simulink model "Model_6DOF_dk"  (R2022a)
settings: Solver=FixedStepAuto  StartTime=0.0  StopTime=Tf  FixedStep=0.05  RelTol=1e-3
InitFcn:
  | run;
StopFcn:
  | save('testdata')
values from neighbouring files (symbols this model uses):
  adap = 1    [run.m]    (also in testdata.mat)
  Ba_0 = [0 0 0 0 0 0]    [run.m]    (also in testdata.mat)
  Bb = 4418825.3321    [testdata.mat]
  Bv_0 = [-5.14444 0 0 0 0 0]    [run.m]    (also in testdata.mat)
  Bx_0 = [0 0 -12 0 0 0]    [run.m]    (also in testdata.mat)
  dA_BP1 = [0.00388591051125 0.00354364911083 0.00553040741788 0.00502167988714 0.0078585088908 0.00748424955325 0.0119232766011 0.0109054787122 0.0168329706434 0.016985509009 0.0156802934897 0.014556760782 ... (616 elements, 616x1)]    [testdata.mat]
  dA_BP2 = [0.00388594063171 0.00354357191533 0.00553040491113 0.00502170939051 0.00785855989083 0.00748435285791 0.0119232653011 0.0109054419481 0.0168329955973 0.0169854794658 0.015680230324 0.0145567225609 ... (616 elements, 616x1)]    [testdata.mat]
  dA_Hull = [0.896301676511 0.898896720864 0.884294141897 0.886832830172 0.870887902011 0.873360353662 0.856223658523 0.858613244346 0.840314828191 0.842595287849 0.823129385532 0.8253007603 ... (2914 elements, 2914x1)]    [testdata.mat]
  dA_PH = [0.00917454029683 0.00917454029683 0.00646521761836 0.00644666811643 0.011728531678 0.0107683420972 0.0165186720105 0.0100399866209 0.0121147162203 0.00917369783051 0.00917369783051 0.00646462373197 ... (550 elements, 550x1)]    [testdata.mat]
  dA_Sail = [0.08073747293 0.0655437895785 0.0678199581962 0.211496702297 0.185444652254 0.10949647106 0.0763960001413 0.0735864235671 0.0440728222699 0.281106392154 0.32735958292 0.104041938486 ... (564 elements, 564x1)]    [testdata.mat]
  dA_SProot = [0.0225345452169 0.0247277274893 0.0225345452169 0.0480467976325 0.0166447079844 0.0410754287554 0.0247277274893 0.0480467976325 0.0468898715351 0.0839833312794 0.0166447079844 0.0255016718 ... (904 elements, 904x1)]    [testdata.mat]
  dA_X1a = [0.0149621011817 0.0166706156701 0.0341149781095 0.0355915100668 0.0512235531199 0.0489176133683 0.0604458424392 0.0503279152264 0.0577124835488 0.0401555322121 0.044833653096 0.0251568218541 ... (200 elements, 200x1)]    [testdata.mat]
  dA_X1b = [0.0149621011817 0.0166706156701 0.0341149781095 0.0355915100668 0.0512235531199 0.0489176133683 0.0604458424392 0.0503279152264 0.0577124835488 0.0401555322121 0.044833653096 0.0251568218541 ... (200 elements, 200x1)]    [testdata.mat]
  dA_X2a = [0.0149620639393 0.0166705502855 0.0341150948266 0.0355913495849 0.051223110376 0.0489180393921 0.0604458270347 0.0503275686692 0.0577128112225 0.0401556683139 0.0448334591683 0.0251566482124 ... (200 elements, 200x1)]    [testdata.mat]
  dA_X2b = [0.0149620639393 0.0166705502855 0.0341150948266 0.0355913495849 0.051223110376 0.0489180393921 0.0604458270347 0.0503275686692 0.0577128112225 0.0401556683139 0.0448334591683 0.0251566482124 ... (200 elements, 200x1)]    [testdata.mat]
  dA_X3a = [0.0149621011817 0.0166706156701 0.0341149781095 0.0355915100668 0.0512235531199 0.0489176133683 0.0604458424392 0.0503279152264 0.0577124835488 0.0401555322121 0.044833653096 0.0251568218541 ... (200 elements, 200x1)]    [testdata.mat]
  dA_X3b = [0.0149621011817 0.0166706156701 0.0341149781095 0.0355915100668 0.0512235531199 0.0489176133683 0.0604458424392 0.0503279152264 0.0577124835488 0.0401555322121 0.044833653096 0.0251568218541 ... (200 elements, 200x1)]    [testdata.mat]
  dA_X4a = [0.0149621011817 0.0166706156701 0.0341149781095 0.0355915100668 0.0512235531199 0.0489176133683 0.0604458424392 0.0503279152264 0.0577124835488 0.0401555322121 0.044833653096 0.0251568218541 ... (200 elements, 200x1)]    [testdata.mat]
  dA_X4b = [0.0149621011817 0.0166706156701 0.0341149781095 0.0355915100668 0.0512235531199 0.0489176133683 0.0604458424392 0.0503279152264 0.0577124835488 0.0401555322121 0.044833653096 0.0251568218541 ... (200 elements, 200x1)]    [testdata.mat]
  Ixx = 52300000    [testdata.mat]
  Ixy = 0    [testdata.mat]
  Ixz = 0    [testdata.mat]
  Iyy = 1375000000    [testdata.mat]
  Iyz = 0    [testdata.mat]
  Izz = 1367000000    [testdata.mat]
  L1 =     [testdata.mat]
  Mb = 4418825.3321    [testdata.mat]
  n_BP1 = [-0.7747315 -0.03638153 -0.4095958 0 -0.1221389 0 -0.01670914 0 0.005209626 0 0.03404154 0 ... (1848 elements, 616x3)]    [testdata.mat]
  n_BP2 = [-0.774731517 -0.0363815315 -0.409595788 0 -0.122138903 0 -0.0167091396 0 0.00520962616 0 0.0340415388 0 ... (1848 elements, 616x3)]    [testdata.mat]
  n_Hull = [-3.334458e-05 -1.700098e-14 -3.354233e-05 -1.686235e-14 -3.289162e-05 -1.685701e-14 -3.291391e-05 -1.698144e-14 -3.338145e-05 -1.688959e-14 -3.29289e-05 -1.682536e-14 ... (8742 elements, 2914x3)]    [testdata.mat]
  n_PH = [0 0 0.01711651 0.01711627 0.2676807 0.2676804 0.7675173 0.7675174 0.9857236 0 0 0.01711456 ... (1650 elements, 550x3)]    [testdata.mat]
  n_Sail = [-0.05126832 -0.05168081 -0.0485872 -0.03288998 -0.03203588 -0.04435105 -0.04335441 -0.04419429 -0.05169604 0.01094904 0.01649325 -0.03825178 ... (1692 elements, 564x3)]    [testdata.mat]
  n_SProot = [-0.7837688 -0.7969784 -0.7837688 -0.79448 -0.280412 -0.3378876 -0.7969784 -0.79448 -0.7910827 -0.3483897 -0.280412 -0.2790298 ... (2712 elements, 904x3)]    [testdata.mat]
  n_X2a = [-0.283297986 -0.283136904 -0.283195704 -0.28313759 -0.2831586 -0.283137113 -0.28313911 -0.283136606 -0.283121586 -0.283136815 -0.283108413 -0.283138901 ... (600 elements, 200x3)]    [testdata.mat]
  n_X2b = [-0.283297986 -0.283136904 -0.283195704 -0.28313759 -0.2831586 -0.283137113 -0.28313911 -0.283136606 -0.283121586 -0.283136815 -0.283108413 -0.283138901 ... (600 elements, 200x3)]    [testdata.mat]
  n_X3a = [-0.283298 -0.2831369 -0.2831957 -0.2831376 -0.2831586 -0.2831371 -0.2831391 -0.2831366 -0.2831216 -0.2831368 -0.2831084 -0.2831389 ... (600 elements, 200x3)]    [testdata.mat]
  n_X4a = [-0.283298 -0.2831369 -0.2831957 -0.2831376 -0.2831586 -0.2831371 -0.2831391 -0.2831366 -0.2831216 -0.2831368 -0.2831084 -0.2831389 ... (600 elements, 200x3)]    [testdata.mat]
  n_X4b = [-0.283298 -0.2831369 -0.2831957 -0.2831376 -0.2831586 -0.2831371 -0.2831391 -0.2831366 -0.2831216 -0.2831368 -0.2831084 -0.2831389 ... (600 elements, 200x3)]    [testdata.mat]
  nt_BP1 = 616    [testdata.mat]
  nt_BP2 = 616    [testdata.mat]
  nt_Hull = 2914    [testdata.mat]
  nt_PH = 550    [testdata.mat]
  nt_Sail = 564    [testdata.mat]
  nt_SProot = 904    [testdata.mat]
  nt_X1a = 200    [testdata.mat]
  nt_X1b = 200    [testdata.mat]
  nt_X2a = 200    [testdata.mat]
  nt_X2b = 200    [testdata.mat]
  nt_X3a = 200    [testdata.mat]
  nt_X3b = 200    [testdata.mat]
  nt_X4a = 200    [testdata.mat]
  nt_X4b = 200    [testdata.mat]
  psi_ref = 0    [run.m]    (also in testdata.mat)
  Seastate = 0    [run.m]    (also in testdata.mat)
  Ts = 0.05    [run.m]    (also in testdata.mat)
  v_ref = Bv_0(1)    [run.m]    (also in testdata.mat = -5.14444)
  vt1_BP1 = [-11.0524049722 -10.9924120522 -10.9924120522 -10.8819663922 -10.8819663922 -10.7297166322 -10.7297166322 -10.5070632922 -10.5070632922 -10.1807245522 -10.1807245522 -9.8815181122 ... (1848 elements, 616x3)]    [testdata.mat]
  vt1_BP2 = [-11.0524048318 -10.9924111396 -10.9924111396 -10.8819658306 -10.8819658306 -10.7297157898 -10.7297157898 -10.5070637134 -10.5070637134 -10.1807238502 -10.1807238502 -9.8815188844 ... (1848 elements, 616x3)]    [testdata.mat]
  vt1_Hull = [3.5122487678 3.7304022878 5.2621803278 5.4863499878 6.9866994878 7.2167238278 8.6832650078 8.9189474678 10.3493567078 10.5904445678 11.9823842078 12.2286247478 ... (8742 elements, 2914x3)]    [testdata.mat]
  vt1_PH = [37.3342788278 37.3342788278 37.4268866678 37.4268866678 37.5892452278 37.5892452278 37.7549453078 37.7549453078 37.8074619278 37.3342788278 37.3342788278 37.4268866678 ... (1650 elements, 550x3)]    [testdata.mat]
  vt1_Sail = [-12.4909433722 -12.1578443722 -12.0399645322 -11.2138368922 -10.6240515922 -11.5111900522 -11.9364967522 -11.6561249722 -12.4909433722 -7.5732648922 -6.8453119522 -11.1890071522 ... (1692 elements, 564x3)]    [testdata.mat]
  vt1_SProot = [29.2099766678 29.1371231078 29.0494854278 29.2099766678 29.2862630078 29.4526510478 29.0494854278 29.1261368078 29.3369263478 29.5706712878 29.0494854278 29.3857364078 ... (2712 elements, 904x3)]    [testdata.mat]
  vt1_X1a = [29.3961751478 29.4776282078 29.4776282078 29.7060309278 29.7060309278 30.0693861278 30.0693861278 30.5458756478 30.5458756478 31.0830460478 31.0830460478 31.6023926678 ... (600 elements, 200x3)]    [testdata.mat]
  vt1_X1b = [29.6638337078 29.6638337078 29.9620713878 29.9620713878 30.3181187678 30.3181187678 30.7116389078 30.7116389078 31.1104380878 31.1104380878 31.4810519678 31.4810519678 ... (600 elements, 200x3)]    [testdata.mat]
  vt1_X2a = [29.3961767624 29.4776272952 29.4776272952 29.7060326828 29.7060326828 30.0693842324 30.0693842324 30.5458736822 30.5458736822 31.083047171 31.083047171 31.6023916148 ... (600 elements, 200x3)]    [testdata.mat]
  vt1_X2b = [29.6638345502 29.6638345502 29.9620708964 29.9620708964 30.3181168022 30.3181168022 30.7116409436 30.7116409436 31.1104372454 31.1104372454 31.4810526698 31.4810526698 ... (600 elements, 200x3)]    [testdata.mat]
  vt1_X3a = [29.3961751478 29.4776282078 29.4776282078 29.7060309278 29.7060309278 30.0693861278 30.0693861278 30.5458756478 30.5458756478 31.0830460478 31.0830460478 31.6023926678 ... (600 elements, 200x3)]    [testdata.mat]
  vt1_X3b = [29.6638337078 29.6638337078 29.9620713878 29.9620713878 30.3181187678 30.3181187678 30.7116389078 30.7116389078 31.1104380878 31.1104380878 31.4810519678 31.4810519678 ... (600 elements, 200x3)]    [testdata.mat]
  vt1_X4a = [29.6638337078 29.6638337078 29.9620713878 29.9620713878 30.3181187678 30.3181187678 30.7116389078 30.7116389078 31.1104380878 31.1104380878 31.4810519678 31.4810519678 ... (600 elements, 200x3)]    [testdata.mat]
  vt1_X4b = [29.3961751478 29.4776282078 29.4776282078 29.7060309278 29.7060309278 30.0693861278 30.0693861278 30.5458756478 30.5458756478 31.0830460478 31.0830460478 31.6023926678 ... (600 elements, 200x3)]    [testdata.mat]
  vt2_BP1 = [-10.9924120522 -10.9494777322 -10.8819663922 -10.8505308322 -10.7297166322 -10.7112259522 -10.5070632922 -10.4997203722 -10.1807245522 -10.1757543922 -9.8815181122 -9.8813004922 ... (1848 elements, 616x3)]    [testdata.mat]
  vt2_BP2 = [-11.0294626294 -11.0294626294 -10.9494786448 -10.9494786448 -10.8505316746 -10.8505316746 -10.7112256012 -10.7112256012 -10.499720302 -10.499720302 -10.1757550942 -10.1757550942 ... (1848 elements, 616x3)]    [testdata.mat]
  vt2_Hull = [1.9517168078 1.9517168078 3.7304022878 3.7304022878 5.4863499878 5.4863499878 7.2167238278 7.2167238278 8.9189474678 8.9189474678 10.5904445678 10.5904445678 ... (8742 elements, 2914x3)]    [testdata.mat]
  vt2_PH = [37.2028433678 37.2028433678 37.3342788278 37.4268866678 37.4268866678 37.5892452278 37.5892452278 37.7549453078 37.7549453078 37.2028433678 37.2028433678 37.3342788278 ... (1650 elements, 550x3)]    [testdata.mat]
  vt2_Sail = [-12.0399645322 -12.0399645322 -11.9364967522 -10.7084881522 -10.7084881522 -12.0399645322 -12.0399645322 -11.9364967522 -12.3734566522 -7.7110323922 -7.7110323922 -11.6561249722 ... (1692 elements, 564x3)]    [testdata.mat]
  vt2_SProot = [29.0494854278 29.0494854278 29.2099766678 29.1261368078 29.0494854278 29.1371231078 29.1371231078 29.2099766678 29.1261368078 29.2099766678 29.2862630078 29.2862630078 ... (2712 elements, 904x3)]    [testdata.mat]
  vt2_X1a = [29.4776282078 29.9620713878 29.7060309278 30.3181187678 30.0693861278 30.7116389078 30.5458756478 31.1104380878 31.0830460478 31.4810519678 31.6023926678 31.7970362078 ... (600 elements, 200x3)]    [testdata.mat]
  vt2_X1b = [29.4776282078 29.9620713878 29.7060309278 30.3181187678 30.0693861278 30.7116389078 30.5458756478 31.1104380878 31.0830460478 31.4810519678 31.6023926678 31.7970362078 ... (600 elements, 200x3)]    [testdata.mat]
  vt2_X2a = [29.6638345502 29.6638345502 29.9620708964 29.9620708964 30.3181168022 30.3181168022 30.7116409436 30.7116409436 31.1104372454 31.1104372454 31.4810526698 31.4810526698 ... (600 elements, 200x3)]    [testdata.mat]
  vt2_X2b = [29.3961767624 29.4776272952 29.4776272952 29.7060326828 29.7060326828 30.0693842324 30.0693842324 30.5458736822 30.5458736822 31.083047171 31.083047171 31.6023916148 ... (600 elements, 200x3)]    [testdata.mat]
  vt2_X3a = [29.4776282078 29.9620713878 29.7060309278 30.3181187678 30.0693861278 30.7116389078 30.5458756478 31.1104380878 31.0830460478 31.4810519678 31.6023926678 31.7970362078 ... (600 elements, 200x3)]    [testdata.mat]
  vt2_X3b = [29.4776282078 29.9620713878 29.7060309278 30.3181187678 30.0693861278 30.7116389078 30.5458756478 31.1104380878 31.0830460478 31.4810519678 31.6023926678 31.7970362078 ... (600 elements, 200x3)]    [testdata.mat]
  vt2_X4a = [29.4776282078 29.9620713878 29.7060309278 30.3181187678 30.0693861278 30.7116389078 30.5458756478 31.1104380878 31.0830460478 31.4810519678 31.6023926678 31.7970362078 ... (600 elements, 200x3)]    [testdata.mat]
  vt2_X4b = [29.4776282078 29.9620713878 29.7060309278 30.3181187678 30.0693861278 30.7116389078 30.5458756478 31.1104380878 31.0830460478 31.4810519678 31.6023926678 31.7970362078 ... (600 elements, 200x3)]    [testdata.mat]
  vt3_BP1 = [-11.0294636122 -11.0294636122 -10.9494777322 -10.9494777322 -10.8505308322 -10.8505308322 -10.7112259522 -10.7112259522 -10.4997203722 -10.4997203722 -10.1757543922 -10.1757543922 ... (1848 elements, 616x3)]    [testdata.mat]
  vt3_BP2 = [-10.9924111396 -10.9494786448 -10.8819658306 -10.8505316746 -10.7297157898 -10.7112256012 -10.5070637134 -10.499720302 -10.1807238502 -10.1757550942 -9.8815188844 -9.8813013346 ... (1848 elements, 616x3)]    [testdata.mat]
  vt3_Hull = [1.7397198278 3.5122487678 3.5122487678 5.2621803278 5.2621803278 6.9866994878 6.9866994878 8.6832650078 8.6832650078 10.3493567078 10.3493567078 11.9823842078 ... (8742 elements, 2914x3)]    [testdata.mat]
  vt3_PH = [37.2028433678 37.3342788278 37.3342788278 37.3342788278 37.4268866678 37.4268866678 37.5892452278 37.5892452278 37.7549453078 37.2028433678 37.3342788278 37.3342788278 ... (1650 elements, 550x3)]    [testdata.mat]
  vt3_Sail = [-12.3734566522 -12.4909433722 -12.3734566522 -11.5111900522 -11.2138368922 -11.7698559922 -11.5111900522 -11.5111900522 -12.1578443722 -8.3109054322 -7.5732648922 -11.5111900522 ... (1692 elements, 564x3)]    [testdata.mat]
  vt3_SProot = [29.1261368078 29.2099766678 29.1261368078 29.3369263478 29.1371231078 29.2099766678 29.2099766678 29.3369263478 29.2548344678 29.3369263478 29.1371231078 29.1371231078 ... (2712 elements, 904x3)]    [testdata.mat]
  vt3_X1a = [29.6638337078 29.6638337078 29.9620713878 29.9620713878 30.3181187678 30.3181187678 30.7116389078 30.7116389078 31.1104380878 31.1104380878 31.4810519678 31.4810519678 ... (600 elements, 200x3)]    [testdata.mat]
  vt3_X1b = [29.3961751478 29.4776282078 29.4776282078 29.7060309278 29.7060309278 30.0693861278 30.0693861278 30.5458756478 30.5458756478 31.0830460478 31.0830460478 31.6023926678 ... (600 elements, 200x3)]    [testdata.mat]
  vt3_X2a = [29.4776272952 29.9620708964 29.7060326828 30.3181168022 30.0693842324 30.7116409436 30.5458736822 31.1104372454 31.083047171 31.4810526698 31.6023916148 31.7970343826 ... (600 elements, 200x3)]    [testdata.mat]
  vt3_X2b = [29.4776272952 29.9620708964 29.7060326828 30.3181168022 30.0693842324 30.7116409436 30.5458736822 31.1104372454 31.083047171 31.4810526698 31.6023916148 31.7970343826 ... (600 elements, 200x3)]    [testdata.mat]
  vt3_X3a = [29.6638337078 29.6638337078 29.9620713878 29.9620713878 30.3181187678 30.3181187678 30.7116389078 30.7116389078 31.1104380878 31.1104380878 31.4810519678 31.4810519678 ... (600 elements, 200x3)]    [testdata.mat]
  vt3_X3b = [29.3961751478 29.4776282078 29.4776282078 29.7060309278 29.7060309278 30.0693861278 30.0693861278 30.5458756478 30.5458756478 31.0830460478 31.0830460478 31.6023926678 ... (600 elements, 200x3)]    [testdata.mat]
  vt3_X4a = [29.3961751478 29.4776282078 29.4776282078 29.7060309278 29.7060309278 30.0693861278 30.0693861278 30.5458756478 30.5458756478 31.0830460478 31.0830460478 31.6023926678 ... (600 elements, 200x3)]    [testdata.mat]
  vt3_X4b = [29.6638337078 29.6638337078 29.9620713878 29.9620713878 30.3181187678 30.3181187678 30.7116389078 30.7116389078 31.1104380878 31.1104380878 31.4810519678 31.4810519678 ... (600 elements, 200x3)]    [testdata.mat]
  Xb = 0    [testdata.mat]
  Xcg = [32.3287332922 0 0]    [testdata.mat]
  Xg = 0    [testdata.mat]
  Yb = 0    [testdata.mat]
  Yg = 0    [testdata.mat]
  z_ref = Bx_0(3)    [run.m]    (also in testdata.mat = -12)
  Zb = 0.4406    [testdata.mat]
  Zg = 0    [testdata.mat]
libraries: simulink x8
(part 6 of 8)

== matlab function Model_6DOF_dk/HDM/HDM B3/Wave, Virtual Mass and Hydrostatic/Wave Particle Motions/Hydrostatic Forces and Moments/X1/MATLAB Function4 ==
  data: time input; Xearth input; Fx_total output; vert1 input; vert2 input; vert3 input; dA input; ntri input; A_wave input; k_wave input; w_wave input; rho input; g input; Fy_total output; Fz_total output; Mx_total output; My_total output; Mz_total output; Zb input; EAX input; dX input; origin input; xcg input
function [Fx_total,Fy_total,Fz_total,Mx_total,My_total,Mz_total]= fcn(time,Xearth,vert1,vert2,vert3,dA,ntri,A_wave,k_wave,w_wave,rho,g,Zb,EAX,dX,origin,xcg)
%EAX=Appendage eulater angle in local coordinate
%its=number of time steps to skip writing grid

x_e=Xearth(1); y_e=Xearth(2); z_e=Xearth(3);
phi=Xearth(4); theta=Xearth(5); psi=Xearth(6);
phiX=EAX(1); thetaX=EAX(2); psiX=EAX(3);


RMat=[cos(theta)*cos(psi) -cos(phi)*sin(psi)+sin(phi)*sin(theta)*cos(psi)  sin(phi)*sin(psi)+cos(phi)*sin(theta)*cos(psi); ...
      cos(theta)*sin(psi)  cos(phi)*cos(psi)+sin(phi)*sin(theta)*sin(psi) -sin(phi)*cos(psi)+cos(phi)*sin(theta)*sin(psi); ...
     -sin(theta)                             sin(phi)*cos(theta)                             cos(phi)*cos(theta)];  
RMATX=[cos(thetaX)*cos(psiX) -cos(phiX)*sin(psiX)+sin(phiX)*sin(thetaX)*cos(psiX)  sin(phiX)*sin(psiX)+cos(phiX)*sin(thetaX)*cos(psiX); ...
      cos(thetaX)*sin(psiX)  cos(phiX)*cos(psiX)+sin(phiX)*sin(thetaX)*sin(psiX) -sin(phiX)*cos(psiX)+cos(phiX)*sin(thetaX)*sin(psiX); ...
     -sin(thetaX)                             sin(phiX)*cos(thetaX)                             cos(phiX)*cos(thetaX)];  
RMATD=[cos(0)*cos(dX) -cos(0)*sin(dX)+sin(0)*sin(0)*cos(dX)  sin(0)*sin(dX)+cos(0)*sin(0)*cos(dX); ...
      cos(0)*sin(dX)  cos(0)*cos(dX)+sin(0)*sin(0)*sin(dX) -sin(0)*cos(dX)+cos(0)*sin(0)*sin(dX); ...
     -sin(0)                             sin(0)*cos(0)                             cos(0)*cos(0)];  


%Rotating the vertices to put in ship coordinate
for i=1:ntri 
    V1=[vert1(i,1); vert1(i,2); vert1(i,3);];
    V2=[vert2(i,1); vert2(i,2); vert2(i,3);];
    V3=[vert3(i,1); vert3(i,2); vert3(i,3);];
        
    %rotating to local z coordinate
    V1_o=inv(RMATX)*(V1-origin*70.2+xcg);
    V2_o=inv(RMATX)*(V2-origin*70.2+xcg);
    V3_o=inv(RMATX)*(V3-origin*70.2+xcg);
    
    %rotating for corresponding appendage deflection
    V1_x=RMATD*V1_o;
    V2_x=RMATD*V2_o;
    V3_x=RMATD*V3_o;
    
        %re-positioning the appendage to local vectors
    V1_r=RMATX*V1_x;
    V2_r=RMATX*V2_x;
    V3_r=RMATX*V3_x;
    
    %re-assigning vertices
    
    for j=1:3
    vert1(i,j)=V1_r(j)+origin(j)*70.2-xcg(j);
    vert2(i,j)=V2_r(j)+origin(j)*70.2-xcg(j);
    vert3(i,j)=V3_r(j)+origin(j)*70.2-xcg(j);
    end  
end

 
%position of mid points in earth coordinate;
mp1=zeros(ntri,3);
mp2=zeros(ntri,3);
mp3=zeros(ntri,3);
nA =zeros(ntri,3);

P1=zeros(ntri,1);
P2=zeros(ntri,1);
P3=zeros(ntri,1);

%position vector of mid points from the CG
r1=zeros(ntri,3);
r2=zeros(ntri,3);
r3=zeros(ntri,3);

v1_w=zeros(ntri,3);
v2_w=zeros(ntri,3);
v3_w=zeros(ntri,3);
n_w=zeros(ntri,3);

%Area of triangle, product of area and unit normal, position vector to each mid-point

for i=1:ntri
    %Area of each triangle
    A=[vert2(i,1)-vert1(i,1); vert2(i,2)-vert1(i,2); vert2(i,3)-vert1(i,3);];
    B=[vert3(i,1)-vert1(i,1); vert3(i,2)-vert1(i,2); vert3(i,3)-vert1(i,3);];
    n=cross(A,B)/norm(cross(A,B));
    C=[n(1); n(2); n(3);];
    %C=[normal(i,1); normal(i,2); normal(i,3);];

    
    %A*n vector calculation
    for j=1:3
        nA(i,j)=dA(i).*C(j);    
    end
    
    %position vector to each mid point of each edge
    for j=1:3
        r1(i,j)=0.5*(vert1(i,j)+vert2(i,j));
        r2(i,j)=0.5*(vert1(i,j)+vert3(i,j));
        r3(i,j)=0.5*(vert2(i,j)+vert3(i,j));
    end
end

%computing mid point location between vertices in earth coordinate
for i=1:ntri
    MP1=RMat*[r1(i,1); r1(i,2); r1(i,3);]+[x_e; y_e; z_e;];
    MP2=RMat*[r2(i,1); r2(i,2); r2(i,3);]+[x_e; y_e; z_e;];
    MP3=RMat*[r3(i,1); r3(i,2); r3(i,3);]+[x_e; y_e; z_e;];
    
    v1i=RMat*[vert1(i,1); vert1(i,2); vert1(i,3);]+[x_e; y_e; z_e;];
    v2i=RMat*[vert2(i,1); vert2(i,2); vert2(i,3);]+[x_e; y_e; z_e;];
    v3i=RMat*[vert3(i,1); vert3(i,2); vert3(i,3);]+[x_e; y_e; z_e;];
    
    for j=1:3
        v1_w(i,j)=v1i(j); v2_w(i,j)=v2i(j); v3_w(i,j)=v3i(j);
        mp1(i,j)=MP1(j);  mp2(i,j)=MP2(j);  mp3(i,j)=MP3(j);
    end
end

for i=1:ntri
    A=[v2_w(i,1)-v1_w(i,1); v2_w(i,2)-v1_w(i,2); v2_w(i,3)-v1_w(i,3);];
    B=[v3_w(i,1)-v1_w(i,1); v3_w(i,2)-v1_w(i,2); v3_w(i,3)-v1_w(i,3);];
    n=cross(A,B)/norm(cross(A,B));
    dA(i,1)=0.5*norm(cross(A,B));
    n_w(i,1)=n(1); n_w(i,2)=n(2); n_w(i,3)=n(3);
end



%computing forces and moments for each triangle
Fx_total=0; Fy_total=0; Fz_total=0;
Mx_total=0; My_total=0; Mz_total=0;

for i=1:ntri
    p1=-rho*g*(mp1(i,3)-A_wave*exp(k_wave.*mp1(i,3)).*sin(k_wave*mp1(i,1)-w_wave.*time));
    p2=-rho*g*(mp2(i,3)-A_wave*exp(k_wave.*mp2(i,3)).*sin(k_wave*mp2(i,1)-w_wave.*time));
    p3=-rho*g*(mp3(i,3)-A_wave*exp(k_wave.*mp3(i,3)).*sin(k_wave*mp3(i,1)-w_wave.*time));
    
    dFx=-nA(i,1)*(p1+p2+p3)./3;
    dFy=-nA(i,2)*(p1+p2+p3)./3;
    dFz=-nA(i,3)*(p1+p2+p3)./3;
    
    dP =-p1.*[r1(i,1); r1(i,2); r1(i,3)-Zb;]...
        -p2.*[r2(i,1); r2(i,2); r2(i,3)-Zb;]...
        -p3.*[r3(i,1); r3(i,2); r3(i,3)-Zb;];
    N =[nA(i,1); nA(i,2); nA(i,3);];
    dM=cross(dP,N);
    Fx_total=Fx_total+dFx;
    Fy_total=Fy_total+dFy;
    Fz_total=Fz_total+dFz;
    Mx_total=Mx_total+dM(1)/3;
    My_total=My_total+dM(2)/3;
    Mz_total=Mz_total+dM(3)/3;
end
end

== matlab function Model_6DOF_dk/HDM/HDM B3/Wave, Virtual Mass and Hydrostatic/Wave Particle Motions/Hydrostatic Forces and Moments/X2/MATLAB Function1 ==
  data: time input; Xearth input; Fx_total output; vert1 input; vert2 input; vert3 input; dA input; ntri input; A_wave input; k_wave input; w_wave input; rho input; g input; Fy_total output; Fz_total output; Mx_total output; My_total output; Mz_total output; Zb input; EAX input; dX input; origin input; xcg input
function [Fx_total,Fy_total,Fz_total,Mx_total,My_total,Mz_total]= fcn(time,Xearth,vert1,vert2,vert3,dA,ntri,A_wave,k_wave,w_wave,rho,g,Zb,EAX,dX,origin,xcg)
%EAX=Appendage eulater angle in local coordinate
%its=number of time steps to skip writing grid

x_e=Xearth(1); y_e=Xearth(2); z_e=Xearth(3);
phi=Xearth(4); theta=Xearth(5); psi=Xearth(6);
phiX=EAX(1); thetaX=EAX(2); psiX=EAX(3);


RMat=[cos(theta)*cos(psi) -cos(phi)*sin(psi)+sin(phi)*sin(theta)*cos(psi)  sin(phi)*sin(psi)+cos(phi)*sin(theta)*cos(psi); ...
      cos(theta)*sin(psi)  cos(phi)*cos(psi)+sin(phi)*sin(theta)*sin(psi) -sin(phi)*cos(psi)+cos(phi)*sin(theta)*sin(psi); ...
     -sin(theta)                             sin(phi)*cos(theta)                             cos(phi)*cos(theta)];  
RMATX=[cos(thetaX)*cos(psiX) -cos(phiX)*sin(psiX)+sin(phiX)*sin(thetaX)*cos(psiX)  sin(phiX)*sin(psiX)+cos(phiX)*sin(thetaX)*cos(psiX); ...
      cos(thetaX)*sin(psiX)  cos(phiX)*cos(psiX)+sin(phiX)*sin(thetaX)*sin(psiX) -sin(phiX)*cos(psiX)+cos(phiX)*sin(thetaX)*sin(psiX); ...
     -sin(thetaX)                             sin(phiX)*cos(thetaX)                             cos(phiX)*cos(thetaX)];  
RMATD=[cos(0)*cos(dX) -cos(0)*sin(dX)+sin(0)*sin(0)*cos(dX)  sin(0)*sin(dX)+cos(0)*sin(0)*cos(dX); ...
      cos(0)*sin(dX)  cos(0)*cos(dX)+sin(0)*sin(0)*sin(dX) -sin(0)*cos(dX)+cos(0)*sin(0)*sin(dX); ...
     -sin(0)                             sin(0)*cos(0)                             cos(0)*cos(0)];  


%Rotating the vertices to put in ship coordinate
for i=1:ntri 
    V1=[vert1(i,1); vert1(i,2); vert1(i,3);];
    V2=[vert2(i,1); vert2(i,2); vert2(i,3);];
    V3=[vert3(i,1); vert3(i,2); vert3(i,3);];
        
    %rotating to local z coordinate
    V1_o=inv(RMATX)*(V1-origin*70.2+xcg);
    V2_o=inv(RMATX)*(V2-origin*70.2+xcg);
    V3_o=inv(RMATX)*(V3-origin*70.2+xcg);
    
    %rotating for corresponding appendage deflection
    V1_x=RMATD*V1_o;
    V2_x=RMATD*V2_o;
    V3_x=RMATD*V3_o;
    
        %re-positioning the appendage to local vectors
    V1_r=RMATX*V1_x;
    V2_r=RMATX*V2_x;
    V3_r=RMATX*V3_x;
    
    %re-assigning vertices
    
    for j=1:3
    vert1(i,j)=V1_r(j)+origin(j)*70.2-xcg(j);
    vert2(i,j)=V2_r(j)+origin(j)*70.2-xcg(j);
    vert3(i,j)=V3_r(j)+origin(j)*70.2-xcg(j);
    end  
end

 
%position of mid points in earth coordinate;
mp1=zeros(ntri,3);
mp2=zeros(ntri,3);
mp3=zeros(ntri,3);
nA =zeros(ntri,3);

P1=zeros(ntri,1);
P2=zeros(ntri,1);
P3=zeros(ntri,1);

%position vector of mid points from the CG
r1=zeros(ntri,3);
r2=zeros(ntri,3);
r3=zeros(ntri,3);

v1_w=zeros(ntri,3);
v2_w=zeros(ntri,3);
v3_w=zeros(ntri,3);
n_w=zeros(ntri,3);

%Area of triangle, product of area and unit normal, position vector to each mid-point

for i=1:ntri
    %Area of each triangle
    A=[vert2(i,1)-vert1(i,1); vert2(i,2)-vert1(i,2); vert2(i,3)-vert1(i,3);];
    B=[vert3(i,1)-vert1(i,1); vert3(i,2)-vert1(i,2); vert3(i,3)-vert1(i,3);];
    n=cross(A,B)/norm(cross(A,B));
    C=[n(1); n(2); n(3);];
    %C=[normal(i,1); normal(i,2); normal(i,3);];

    
    %A*n vector calculation
    for j=1:3
        nA(i,j)=dA(i).*C(j);    
    end
    
    %position vector to each mid point of each edge
    for j=1:3
        r1(i,j)=0.5*(vert1(i,j)+vert2(i,j));
        r2(i,j)=0.5*(vert1(i,j)+vert3(i,j));
        r3(i,j)=0.5*(vert2(i,j)+vert3(i,j));
    end
end

%computing mid point location between vertices in earth coordinate
for i=1:ntri
    MP1=RMat*[r1(i,1); r1(i,2); r1(i,3);]+[x_e; y_e; z_e;];
    MP2=RMat*[r2(i,1); r2(i,2); r2(i,3);]+[x_e; y_e; z_e;];
    MP3=RMat*[r3(i,1); r3(i,2); r3(i,3);]+[x_e; y_e; z_e;];
    
    v1i=RMat*[vert1(i,1); vert1(i,2); vert1(i,3);]+[x_e; y_e; z_e;];
    v2i=RMat*[vert2(i,1); vert2(i,2); vert2(i,3);]+[x_e; y_e; z_e;];
    v3i=RMat*[vert3(i,1); vert3(i,2); vert3(i,3);]+[x_e; y_e; z_e;];
    
    for j=1:3
        v1_w(i,j)=v1i(j); v2_w(i,j)=v2i(j); v3_w(i,j)=v3i(j);
        mp1(i,j)=MP1(j);  mp2(i,j)=MP2(j);  mp3(i,j)=MP3(j);
    end
end

for i=1:ntri
    A=[v2_w(i,1)-v1_w(i,1); v2_w(i,2)-v1_w(i,2); v2_w(i,3)-v1_w(i,3);];
    B=[v3_w(i,1)-v1_w(i,1); v3_w(i,2)-v1_w(i,2); v3_w(i,3)-v1_w(i,3);];
    n=cross(A,B)/norm(cross(A,B));
    dA(i,1)=0.5*norm(cross(A,B));
    n_w(i,1)=n(1); n_w(i,2)=n(2); n_w(i,3)=n(3);
end


%computing forces and moments for each triangle
Fx_total=0; Fy_total=0; Fz_total=0;
Mx_total=0; My_total=0; Mz_total=0;

for i=1:ntri
    p1=-rho*g*(mp1(i,3)-A_wave*exp(k_wave.*mp1(i,3)).*sin(k_wave*mp1(i,1)-w_wave.*time));
    p2=-rho*g*(mp2(i,3)-A_wave*exp(k_wave.*mp2(i,3)).*sin(k_wave*mp2(i,1)-w_wave.*time));
    p3=-rho*g*(mp3(i,3)-A_wave*exp(k_wave.*mp3(i,3)).*sin(k_wave*mp3(i,1)-w_wave.*time));
    
    dFx=-nA(i,1)*(p1+p2+p3)./3;
    dFy=-nA(i,2)*(p1+p2+p3)./3;
    dFz=-nA(i,3)*(p1+p2+p3)./3;
    
    dP =-p1.*[r1(i,1); r1(i,2); r1(i,3)-Zb;]...
        -p2.*[r2(i,1); r2(i,2); r2(i,3)-Zb;]...
        -p3.*[r3(i,1); r3(i,2); r3(i,3)-Zb;];
    N =[nA(i,1); nA(i,2); nA(i,3);];
    dM=cross(dP,N);
    Fx_total=Fx_total+dFx;
    Fy_total=Fy_total+dFy;
    Fz_total=Fz_total+dFz;
    Mx_total=Mx_total+dM(1)/3;
    My_total=My_total+dM(2)/3;
    Mz_total=Mz_total+dM(3)/3;
end
end

== matlab function Model_6DOF_dk/HDM/HDM B3/Wave, Virtual Mass and Hydrostatic/Wave Particle Motions/Hydrostatic Forces and Moments/X2/MATLAB Function4 ==
  data: time input; Xearth input; Fx_total output; vert1 input; vert2 input; vert3 input; dA input; ntri input; A_wave input; k_wave input; w_wave input; rho input; g input; Fy_total output; Fz_total output; Mx_total output; My_total output; Mz_total output; Zb input; EAX input; dX input; origin input; xcg input
function [Fx_total,Fy_total,Fz_total,Mx_total,My_total,Mz_total]= fcn(time,Xearth,vert1,vert2,vert3,dA,ntri,A_wave,k_wave,w_wave,rho,g,Zb,EAX,dX,origin,xcg)
%EAX=Appendage eulater angle in local coordinate
%its=number of time steps to skip writing grid

x_e=Xearth(1); y_e=Xearth(2); z_e=Xearth(3);
phi=Xearth(4); theta=Xearth(5); psi=Xearth(6);
phiX=EAX(1); thetaX=EAX(2); psiX=EAX(3);


RMat=[cos(theta)*cos(psi) -cos(phi)*sin(psi)+sin(phi)*sin(theta)*cos(psi)  sin(phi)*sin(psi)+cos(phi)*sin(theta)*cos(psi); ...
      cos(theta)*sin(psi)  cos(phi)*cos(psi)+sin(phi)*sin(theta)*sin(psi) -sin(phi)*cos(psi)+cos(phi)*sin(theta)*sin(psi); ...
     -sin(theta)                             sin(phi)*cos(theta)                             cos(phi)*cos(theta)];  
RMATX=[cos(thetaX)*cos(psiX) -cos(phiX)*sin(psiX)+sin(phiX)*sin(thetaX)*cos(psiX)  sin(phiX)*sin(psiX)+cos(phiX)*sin(thetaX)*cos(psiX); ...
      cos(thetaX)*sin(psiX)  cos(phiX)*cos(psiX)+sin(phiX)*sin(thetaX)*sin(psiX) -sin(phiX)*cos(psiX)+cos(phiX)*sin(thetaX)*sin(psiX); ...
     -sin(thetaX)                             sin(phiX)*cos(thetaX)                             cos(phiX)*cos(thetaX)];  
RMATD=[cos(0)*cos(dX) -cos(0)*sin(dX)+sin(0)*sin(0)*cos(dX)  sin(0)*sin(dX)+cos(0)*sin(0)*cos(dX); ...
      cos(0)*sin(dX)  cos(0)*cos(dX)+sin(0)*sin(0)*sin(dX) -sin(0)*cos(dX)+cos(0)*sin(0)*sin(dX); ...
     -sin(0)                             sin(0)*cos(0)                             cos(0)*cos(0)];  


%Rotating the vertices to put in ship coordinate
for i=1:ntri 
    V1=[vert1(i,1); vert1(i,2); vert1(i,3);];
    V2=[vert2(i,1); vert2(i,2); vert2(i,3);];
    V3=[vert3(i,1); vert3(i,2); vert3(i,3);];
        
    %rotating to local z coordinate
    V1_o=inv(RMATX)*(V1-origin*70.2+xcg);
    V2_o=inv(RMATX)*(V2-origin*70.2+xcg);
    V3_o=inv(RMATX)*(V3-origin*70.2+xcg);
    
    %rotating for corresponding appendage deflection
    V1_x=RMATD*V1_o;
    V2_x=RMATD*V2_o;
    V3_x=RMATD*V3_o;
    
        %re-positioning the appendage to local vectors
    V1_r=RMATX*V1_x;
    V2_r=RMATX*V2_x;
    V3_r=RMATX*V3_x;
    
    %re-assigning vertices
    
    for j=1:3
    vert1(i,j)=V1_r(j)+origin(j)*70.2-xcg(j);
    vert2(i,j)=V2_r(j)+origin(j)*70.2-xcg(j);
    vert3(i,j)=V3_r(j)+origin(j)*70.2-xcg(j);
    end  
end

 
%position of mid points in earth coordinate;
mp1=zeros(ntri,3);
mp2=zeros(ntri,3);
mp3=zeros(ntri,3);
nA =zeros(ntri,3);

P1=zeros(ntri,1);
P2=zeros(ntri,1);
P3=zeros(ntri,1);

%position vector of mid points from the CG
r1=zeros(ntri,3);
r2=zeros(ntri,3);
r3=zeros(ntri,3);

v1_w=zeros(ntri,3);
v2_w=zeros(ntri,3);
v3_w=zeros(ntri,3);
n_w=zeros(ntri,3);

%Area of triangle, product of area and unit normal, position vector to each mid-point

for i=1:ntri
    %Area of each triangle
    A=[vert2(i,1)-vert1(i,1); vert2(i,2)-vert1(i,2); vert2(i,3)-vert1(i,3);];
    B=[vert3(i,1)-vert1(i,1); vert3(i,2)-vert1(i,2); vert3(i,3)-vert1(i,3);];
    n=cross(A,B)/norm(cross(A,B));
    C=[n(1); n(2); n(3);];
    %C=[normal(i,1); normal(i,2); normal(i,3);];

    
    %A*n vector calculation
    for j=1:3
        nA(i,j)=dA(i).*C(j);    
    end
    
    %position vector to each mid point of each edge
    for j=1:3
        r1(i,j)=0.5*(vert1(i,j)+vert2(i,j));
        r2(i,j)=0.5*(vert1(i,j)+vert3(i,j));
        r3(i,j)=0.5*(vert2(i,j)+vert3(i,j));
    end
end

%computing mid point location between vertices in earth coordinate
for i=1:ntri
    MP1=RMat*[r1(i,1); r1(i,2); r1(i,3);]+[x_e; y_e; z_e;];
    MP2=RMat*[r2(i,1); r2(i,2); r2(i,3);]+[x_e; y_e; z_e;];
    MP3=RMat*[r3(i,1); r3(i,2); r3(i,3);]+[x_e; y_e; z_e;];
    
    v1i=RMat*[vert1(i,1); vert1(i,2); vert1(i,3);]+[x_e; y_e; z_e;];
    v2i=RMat*[vert2(i,1); vert2(i,2); vert2(i,3);]+[x_e; y_e; z_e;];
    v3i=RMat*[vert3(i,1); vert3(i,2); vert3(i,3);]+[x_e; y_e; z_e;];
    
    for j=1:3
        v1_w(i,j)=v1i(j); v2_w(i,j)=v2i(j); v3_w(i,j)=v3i(j);
        mp1(i,j)=MP1(j);  mp2(i,j)=MP2(j);  mp3(i,j)=MP3(j);
    end
end

for i=1:ntri
    A=[v2_w(i,1)-v1_w(i,1); v2_w(i,2)-v1_w(i,2); v2_w(i,3)-v1_w(i,3);];
    B=[v3_w(i,1)-v1_w(i,1); v3_w(i,2)-v1_w(i,2); v3_w(i,3)-v1_w(i,3);];
    n=cross(A,B)/norm(cross(A,B));
    dA(i,1)=0.5*norm(cross(A,B));
    n_w(i,1)=n(1); n_w(i,2)=n(2); n_w(i,3)=n(3);
end



%computing forces and moments for each triangle
Fx_total=0; Fy_total=0; Fz_total=0;
Mx_total=0; My_total=0; Mz_total=0;

for i=1:ntri
    p1=-rho*g*(mp1(i,3)-A_wave*exp(k_wave.*mp1(i,3)).*sin(k_wave*mp1(i,1)-w_wave.*time));
    p2=-rho*g*(mp2(i,3)-A_wave*exp(k_wave.*mp2(i,3)).*sin(k_wave*mp2(i,1)-w_wave.*time));
    p3=-rho*g*(mp3(i,3)-A_wave*exp(k_wave.*mp3(i,3)).*sin(k_wave*mp3(i,1)-w_wave.*time));
    
    dFx=-nA(i,1)*(p1+p2+p3)./3;
    dFy=-nA(i,2)*(p1+p2+p3)./3;
    dFz=-nA(i,3)*(p1+p2+p3)./3;
    
    dP =-p1.*[r1(i,1); r1(i,2); r1(i,3)-Zb;]...
        -p2.*[r2(i,1); r2(i,2); r2(i,3)-Zb;]...
        -p3.*[r3(i,1); r3(i,2); r3(i,3)-Zb;];
    N =[nA(i,1); nA(i,2); nA(i,3);];
    dM=cross(dP,N);
    Fx_total=Fx_total+dFx;
    Fy_total=Fy_total+dFy;
    Fz_total=Fz_total+dFz;
    Mx_total=Mx_total+dM(1)/3;
    My_total=My_total+dM(2)/3;
    Mz_total=Mz_total+dM(3)/3;
end
end

== matlab function Model_6DOF_dk/HDM/HDM B3/Wave, Virtual Mass and Hydrostatic/Wave Particle Motions/Hydrostatic Forces and Moments/X3/MATLAB Function1 ==
  data: time input; Xearth input; Fx_total output; vert1 input; vert2 input; vert3 input; dA input; ntri input; A_wave input; k_wave input; w_wave input; rho input; g input; Fy_total output; Fz_total output; Mx_total output; My_total output; Mz_total output; Zb input; EAX input; dX input; origin input; xcg input
function [Fx_total,Fy_total,Fz_total,Mx_total,My_total,Mz_total]= fcn(time,Xearth,vert1,vert2,vert3,dA,ntri,A_wave,k_wave,w_wave,rho,g,Zb,EAX,dX,origin,xcg)
%EAX=Appendage eulater angle in local coordinate
%its=number of time steps to skip writing grid

x_e=Xearth(1); y_e=Xearth(2); z_e=Xearth(3);
phi=Xearth(4); theta=Xearth(5); psi=Xearth(6);
phiX=EAX(1); thetaX=EAX(2); psiX=EAX(3);


RMat=[cos(theta)*cos(psi) -cos(phi)*sin(psi)+sin(phi)*sin(theta)*cos(psi)  sin(phi)*sin(psi)+cos(phi)*sin(theta)*cos(psi); ...
      cos(theta)*sin(psi)  cos(phi)*cos(psi)+sin(phi)*sin(theta)*sin(psi) -sin(phi)*cos(psi)+cos(phi)*sin(theta)*sin(psi); ...
     -sin(theta)                             sin(phi)*cos(theta)                             cos(phi)*cos(theta)];  
RMATX=[cos(thetaX)*cos(psiX) -cos(phiX)*sin(psiX)+sin(phiX)*sin(thetaX)*cos(psiX)  sin(phiX)*sin(psiX)+cos(phiX)*sin(thetaX)*cos(psiX); ...
      cos(thetaX)*sin(psiX)  cos(phiX)*cos(psiX)+sin(phiX)*sin(thetaX)*sin(psiX) -sin(phiX)*cos(psiX)+cos(phiX)*sin(thetaX)*sin(psiX); ...
     -sin(thetaX)                             sin(phiX)*cos(thetaX)                             cos(phiX)*cos(thetaX)];  
RMATD=[cos(0)*cos(dX) -cos(0)*sin(dX)+sin(0)*sin(0)*cos(dX)  sin(0)*sin(dX)+cos(0)*sin(0)*cos(dX); ...
      cos(0)*sin(dX)  cos(0)*cos(dX)+sin(0)*sin(0)*sin(dX) -sin(0)*cos(dX)+cos(0)*sin(0)*sin(dX); ...
     -sin(0)                             sin(0)*cos(0)                             cos(0)*cos(0)];  


%Rotating the vertices to put in ship coordinate
for i=1:ntri 
    V1=[vert1(i,1); vert1(i,2); vert1(i,3);];
    V2=[vert2(i,1); vert2(i,2); vert2(i,3);];
    V3=[vert3(i,1); vert3(i,2); vert3(i,3);];
        
    %rotating to local z coordinate
    V1_o=inv(RMATX)*(V1-origin*70.2+xcg);
    V2_o=inv(RMATX)*(V2-origin*70.2+xcg);
    V3_o=inv(RMATX)*(V3-origin*70.2+xcg);
    
    %rotating for corresponding appendage deflection
    V1_x=RMATD*V1_o;
    V2_x=RMATD*V2_o;
    V3_x=RMATD*V3_o;
    
        %re-positioning the appendage to local vectors
    V1_r=RMATX*V1_x;
    V2_r=RMATX*V2_x;
    V3_r=RMATX*V3_x;
    
    %re-assigning vertices
    
    for j=1:3
    vert1(i,j)=V1_r(j)+origin(j)*70.2-xcg(j);
    vert2(i,j)=V2_r(j)+origin(j)*70.2-xcg(j);
    vert3(i,j)=V3_r(j)+origin(j)*70.2-xcg(j);
    end  
end

 
%position of mid points in earth coordinate;
mp1=zeros(ntri,3);
mp2=zeros(ntri,3);
mp3=zeros(ntri,3);
nA =zeros(ntri,3);

P1=zeros(ntri,1);
P2=zeros(ntri,1);
P3=zeros(ntri,1);

%position vector of mid points from the CG
r1=zeros(ntri,3);
r2=zeros(ntri,3);
r3=zeros(ntri,3);

v1_w=zeros(ntri,3);
v2_w=zeros(ntri,3);
v3_w=zeros(ntri,3);
n_w=zeros(ntri,3);

%Area of triangle, product of area and unit normal, position vector to each mid-point

for i=1:ntri
    %Area of each triangle
    A=[vert2(i,1)-vert1(i,1); vert2(i,2)-vert1(i,2); vert2(i,3)-vert1(i,3);];
    B=[vert3(i,1)-vert1(i,1); vert3(i,2)-vert1(i,2); vert3(i,3)-vert1(i,3);];
    n=cross(A,B)/norm(cross(A,B));
    C=[n(1); n(2); n(3);];
    %C=[normal(i,1); normal(i,2); normal(i,3);];

    
    %A*n vector calculation
    for j=1:3
        nA(i,j)=dA(i).*C(j);    
    end
    
    %position vector to each mid point of each edge
    for j=1:3
        r1(i,j)=0.5*(vert1(i,j)+vert2(i,j));
        r2(i,j)=0.5*(vert1(i,j)+vert3(i,j));
        r3(i,j)=0.5*(vert2(i,j)+vert3(i,j));
    end
end

%computing mid point location between vertices in earth coordinate
for i=1:ntri
    MP1=RMat*[r1(i,1); r1(i,2); r1(i,3);]+[x_e; y_e; z_e;];
    MP2=RMat*[r2(i,1); r2(i,2); r2(i,3);]+[x_e; y_e; z_e;];
    MP3=RMat*[r3(i,1); r3(i,2); r3(i,3);]+[x_e; y_e; z_e;];
    
    v1i=RMat*[vert1(i,1); vert1(i,2); vert1(i,3);]+[x_e; y_e; z_e;];
    v2i=RMat*[vert2(i,1); vert2(i,2); vert2(i,3);]+[x_e; y_e; z_e;];
    v3i=RMat*[vert3(i,1); vert3(i,2); vert3(i,3);]+[x_e; y_e; z_e;];
    
    for j=1:3
        v1_w(i,j)=v1i(j); v2_w(i,j)=v2i(j); v3_w(i,j)=v3i(j);
        mp1(i,j)=MP1(j);  mp2(i,j)=MP2(j);  mp3(i,j)=MP3(j);
    end
end

for i=1:ntri
    A=[v2_w(i,1)-v1_w(i,1); v2_w(i,2)-v1_w(i,2); v2_w(i,3)-v1_w(i,3);];
    B=[v3_w(i,1)-v1_w(i,1); v3_w(i,2)-v1_w(i,2); v3_w(i,3)-v1_w(i,3);];
    n=cross(A,B)/norm(cross(A,B));
    dA(i,1)=0.5*norm(cross(A,B));
    n_w(i,1)=n(1); n_w(i,2)=n(2); n_w(i,3)=n(3);
end



%computing forces and moments for each triangle
Fx_total=0; Fy_total=0; Fz_total=0;
Mx_total=0; My_total=0; Mz_total=0;

for i=1:ntri
    p1=-rho*g*(mp1(i,3)-A_wave*exp(k_wave.*mp1(i,3)).*sin(k_wave*mp1(i,1)-w_wave.*time));
    p2=-rho*g*(mp2(i,3)-A_wave*exp(k_wave.*mp2(i,3)).*sin(k_wave*mp2(i,1)-w_wave.*time));
    p3=-rho*g*(mp3(i,3)-A_wave*exp(k_wave.*mp3(i,3)).*sin(k_wave*mp3(i,1)-w_wave.*time));
    
    dFx=-nA(i,1)*(p1+p2+p3)./3;
    dFy=-nA(i,2)*(p1+p2+p3)./3;
    dFz=-nA(i,3)*(p1+p2+p3)./3;
    
    dP =-p1.*[r1(i,1); r1(i,2); r1(i,3)-Zb;]...
        -p2.*[r2(i,1); r2(i,2); r2(i,3)-Zb;]...
        -p3.*[r3(i,1); r3(i,2); r3(i,3)-Zb;];
    N =[nA(i,1); nA(i,2); nA(i,3);];
    dM=cross(dP,N);
    Fx_total=Fx_total+dFx;
    Fy_total=Fy_total+dFy;
    Fz_total=Fz_total+dFz;
    Mx_total=Mx_total+dM(1)/3;
    My_total=My_total+dM(2)/3;
    Mz_total=Mz_total+dM(3)/3;
end
end

== matlab function Model_6DOF_dk/HDM/HDM B3/Wave, Virtual Mass and Hydrostatic/Wave Particle Motions/Hydrostatic Forces and Moments/X3/MATLAB Function4 ==
  data: time input; Xearth input; Fx_total output; vert1 input; vert2 input; vert3 input; dA input; ntri input; A_wave input; k_wave input; w_wave input; rho input; g input; Fy_total output; Fz_total output; Mx_total output; My_total output; Mz_total output; Zb input; EAX input; dX input; origin input; xcg input
function [Fx_total,Fy_total,Fz_total,Mx_total,My_total,Mz_total]= fcn(time,Xearth,vert1,vert2,vert3,dA,ntri,A_wave,k_wave,w_wave,rho,g,Zb,EAX,dX,origin,xcg)
%EAX=Appendage eulater angle in local coordinate
%its=number of time steps to skip writing grid

x_e=Xearth(1); y_e=Xearth(2); z_e=Xearth(3);
phi=Xearth(4); theta=Xearth(5); psi=Xearth(6);
phiX=EAX(1); thetaX=EAX(2); psiX=EAX(3);


RMat=[cos(theta)*cos(psi) -cos(phi)*sin(psi)+sin(phi)*sin(theta)*cos(psi)  sin(phi)*sin(psi)+cos(phi)*sin(theta)*cos(psi); ...
      cos(theta)*sin(psi)  cos(phi)*cos(psi)+sin(phi)*sin(theta)*sin(psi) -sin(phi)*cos(psi)+cos(phi)*sin(theta)*sin(psi); ...
     -sin(theta)                             sin(phi)*cos(theta)                             cos(phi)*cos(theta)];  
RMATX=[cos(thetaX)*cos(psiX) -cos(phiX)*sin(psiX)+sin(phiX)*sin(thetaX)*cos(psiX)  sin(phiX)*sin(psiX)+cos(phiX)*sin(thetaX)*cos(psiX); ...
      cos(thetaX)*sin(psiX)  cos(phiX)*cos(psiX)+sin(phiX)*sin(thetaX)*sin(psiX) -sin(phiX)*cos(psiX)+cos(phiX)*sin(thetaX)*sin(psiX); ...
     -sin(thetaX)                             sin(phiX)*cos(thetaX)                             cos(phiX)*cos(thetaX)];  
RMATD=[cos(0)*cos(dX) -cos(0)*sin(dX)+sin(0)*sin(0)*cos(dX)  sin(0)*sin(dX)+cos(0)*sin(0)*cos(dX); ...
      cos(0)*sin(dX)  cos(0)*cos(dX)+sin(0)*sin(0)*sin(dX) -sin(0)*cos(dX)+cos(0)*sin(0)*sin(dX); ...
     -sin(0)                             sin(0)*cos(0)                             cos(0)*cos(0)];  


%Rotating the vertices to put in ship coordinate
for i=1:ntri 
    V1=[vert1(i,1); vert1(i,2); vert1(i,3);];
    V2=[vert2(i,1); vert2(i,2); vert2(i,3);];
    V3=[vert3(i,1); vert3(i,2); vert3(i,3);];
        
    %rotating to local z coordinate
    V1_o=inv(RMATX)*(V1-origin*70.2+xcg);
    V2_o=inv(RMATX)*(V2-origin*70.2+xcg);
    V3_o=inv(RMATX)*(V3-origin*70.2+xcg);
    
    %rotating for corresponding appendage deflection
    V1_x=RMATD*V1_o;
    V2_x=RMATD*V2_o;
    V3_x=RMATD*V3_o;
    
        %re-positioning the appendage to local vectors
    V1_r=RMATX*V1_x;
    V2_r=RMATX*V2_x;
    V3_r=RMATX*V3_x;
    
    %re-assigning vertices
    
    for j=1:3
    vert1(i,j)=V1_r(j)+origin(j)*70.2-xcg(j);
    vert2(i,j)=V2_r(j)+origin(j)*70.2-xcg(j);
    vert3(i,j)=V3_r(j)+origin(j)*70.2-xcg(j);
    end  
end

 
%position of mid points in earth coordinate;
mp1=zeros(ntri,3);
mp2=zeros(ntri,3);
mp3=zeros(ntri,3);
nA =zeros(ntri,3);

P1=zeros(ntri,1);
P2=zeros(ntri,1);
P3=zeros(ntri,1);

%position vector of mid points from the CG
r1=zeros(ntri,3);
r2=zeros(ntri,3);
r3=zeros(ntri,3);

v1_w=zeros(ntri,3);
v2_w=zeros(ntri,3);
v3_w=zeros(ntri,3);
n_w=zeros(ntri,3);

%Area of triangle, product of area and unit normal, position vector to each mid-point

for i=1:ntri
    %Area of each triangle
    A=[vert2(i,1)-vert1(i,1); vert2(i,2)-vert1(i,2); vert2(i,3)-vert1(i,3);];
    B=[vert3(i,1)-vert1(i,1); vert3(i,2)-vert1(i,2); vert3(i,3)-vert1(i,3);];
    n=cross(A,B)/norm(cross(A,B));
    C=[n(1); n(2); n(3);];
    %C=[normal(i,1); normal(i,2); normal(i,3);];

    
    %A*n vector calculation
    for j=1:3
        nA(i,j)=dA(i).*C(j);    
    end
    
    %position vector to each mid point of each edge
    for j=1:3
        r1(i,j)=0.5*(vert1(i,j)+vert2(i,j));
        r2(i,j)=0.5*(vert1(i,j)+vert3(i,j));
        r3(i,j)=0.5*(vert2(i,j)+vert3(i,j));
    end
end

%computing mid point location between vertices in earth coordinate
for i=1:ntri
    MP1=RMat*[r1(i,1); r1(i,2); r1(i,3);]+[x_e; y_e; z_e;];
    MP2=RMat*[r2(i,1); r2(i,2); r2(i,3);]+[x_e; y_e; z_e;];
    MP3=RMat*[r3(i,1); r3(i,2); r3(i,3);]+[x_e; y_e; z_e;];
    
    v1i=RMat*[vert1(i,1); vert1(i,2); vert1(i,3);]+[x_e; y_e; z_e;];
    v2i=RMat*[vert2(i,1); vert2(i,2); vert2(i,3);]+[x_e; y_e; z_e;];
    v3i=RMat*[vert3(i,1); vert3(i,2); vert3(i,3);]+[x_e; y_e; z_e;];
    
    for j=1:3
        v1_w(i,j)=v1i(j); v2_w(i,j)=v2i(j); v3_w(i,j)=v3i(j);
        mp1(i,j)=MP1(j);  mp2(i,j)=MP2(j);  mp3(i,j)=MP3(j);
    end
end

for i=1:ntri
    A=[v2_w(i,1)-v1_w(i,1); v2_w(i,2)-v1_w(i,2); v2_w(i,3)-v1_w(i,3);];
    B=[v3_w(i,1)-v1_w(i,1); v3_w(i,2)-v1_w(i,2); v3_w(i,3)-v1_w(i,3);];
    n=cross(A,B)/norm(cross(A,B));
    dA(i,1)=0.5*norm(cross(A,B));
    n_w(i,1)=n(1); n_w(i,2)=n(2); n_w(i,3)=n(3);
end



%computing forces and moments for each triangle
Fx_total=0; Fy_total=0; Fz_total=0;
Mx_total=0; My_total=0; Mz_total=0;

for i=1:ntri
    p1=-rho*g*(mp1(i,3)-A_wave*exp(k_wave.*mp1(i,3)).*sin(k_wave*mp1(i,1)-w_wave.*time));
    p2=-rho*g*(mp2(i,3)-A_wave*exp(k_wave.*mp2(i,3)).*sin(k_wave*mp2(i,1)-w_wave.*time));
    p3=-rho*g*(mp3(i,3)-A_wave*exp(k_wave.*mp3(i,3)).*sin(k_wave*mp3(i,1)-w_wave.*time));
    
    dFx=-nA(i,1)*(p1+p2+p3)./3;
    dFy=-nA(i,2)*(p1+p2+p3)./3;
    dFz=-nA(i,3)*(p1+p2+p3)./3;
    
    dP =-p1.*[r1(i,1); r1(i,2); r1(i,3)-Zb;]...
        -p2.*[r2(i,1); r2(i,2); r2(i,3)-Zb;]...
        -p3.*[r3(i,1); r3(i,2); r3(i,3)-Zb;];
    N =[nA(i,1); nA(i,2); nA(i,3);];
    dM=cross(dP,N);
    Fx_total=Fx_total+dFx;
    Fy_total=Fy_total+dFy;
    Fz_total=Fz_total+dFz;
    Mx_total=Mx_total+dM(1)/3;
    My_total=My_total+dM(2)/3;
    Mz_total=Mz_total+dM(3)/3;
end
end
